simulink model "Theta1model"  (R2020a)
settings: Solver=VariableStepAuto  StartTime=0.0  StopTime=10.0  RelTol=1e-3
settings Model: Creator=marce  LastModifiedBy=marce

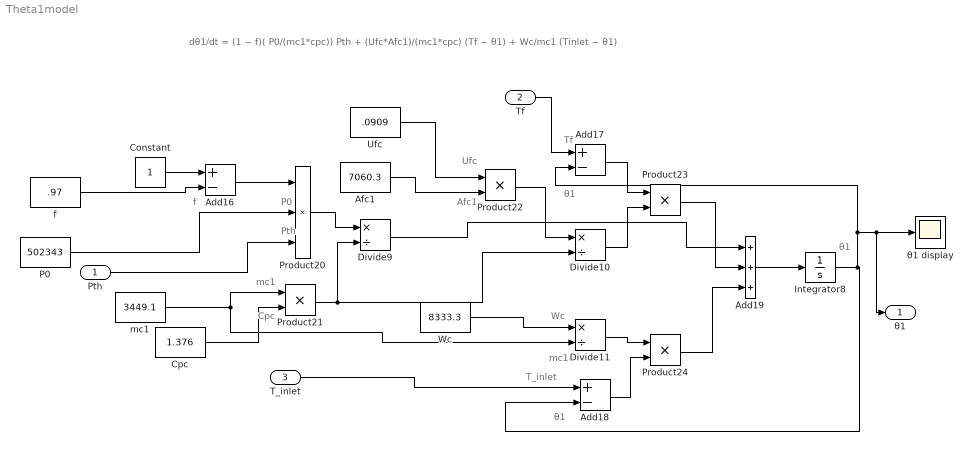
== system Theta1model ==
  note: dθ1/dt = (1 − f)( P0/(mc1*cpc)) Pth + (Ufc*Afc1)/(mc1*cpc) (Tf − θ1) + Wc/mc1 (Tinlet − θ1)
  note: T_inlet
  note: θ1
  note: θ1
  note: mc1
  note: Afc1
  note: mc1
  note: Tf
  note: Pth
  note: Ufc
  note: P0
  note: Cpc
  note: f
  note: Wc
  note: θ1
  Pth : Inport
  Tf : Inport  Port=2
  T_inlet : Inport  Port=3
  Add16 : Sum  Inputs=+-
  Add17 : Sum  Inputs=+-
  Add18 : Sum  Inputs=+-
  Add19 : Sum  Inputs=+++
  Afc1 : Constant  Value=7060.3
  Constant : Constant
  Cpc : Constant  Value=1.376
  Divide10 : Product  Inputs=*/
  Divide11 : Product  Inputs=*/
  Divide9 : Product  Inputs=*/
  Integrator8 : Integrator
  P0 : Constant  Value=502343
  Product20 : Product  Inputs=3
  Product{21..24} (4 alike) : Product
  Ufc : Constant  Value=.0909
  Wc : Constant  Value=8333.3
  f : Constant  Value=.97
  mc1 : Constant  Value=3449.1
  θ1 display : Scope
  θ1 : Outport
  wires:
  Integrator8/1 -> θ1/1, θ1 display/1, Add17/2, Add18/2
  Product21/1 -> Divide10/2, Divide9/2
  Product24/1 -> Add19/3
  Product23/1 -> Add19/2
  Divide10/1 -> Product23/2
  Add19/1 -> Integrator8/1
  Divide11/1 -> Product24/1
  Add18/1 -> Product24/2
  Product22/1 -> Divide10/1
  Product20/1 -> Divide9/1
  Constant/1 -> Add16/1
  Divide9/1 -> Add19/1
  Add16/1 -> Product20/1
  Add17/1 -> Product23/1
  f/1 -> Add16/2
  P0/1 -> Product20/2
  Pth/1 -> Product20/3
  mc1/1 -> Product21/1, Divide11/2
  Cpc/1 -> Product21/2
  T_inlet/1 -> Add18/1
  Wc/1 -> Divide11/1
  Ufc/1 -> Product22/1
  Afc1/1 -> Product22/2
  Tf/1 -> Add17/1
